simulink model "Variant1"  (R2021a)
settings: Solver=FixedStepAuto  StartTime=0.0  StopTime=STime  FixedStep=1e-3  RelTol=1e-3
undefined symbols (not defined in the file): C, J, Kp, Mc, Ra, Ta, Tp, Uc
settings Model: Creator=akangmufti  LastModifiedBy=akangmufti

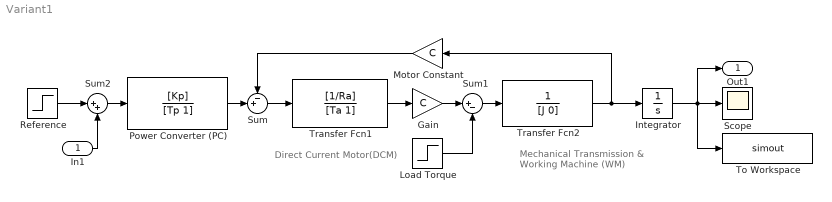
== system Variant1 ==
  note: Direct Current Motor(DCM)
  note: Mechanical Transmission &
      | Working Machine (WM)
  In1 : Inport
  Gain : Gain  Gain=C
  Integrator : Integrator  ContinuousStateAttributes='AngularPosition'
  Load Torque : Step  After=Mc  SampleTime=0
  Motor Constant : Gain  Gain=C
  Power Converter (PC) : TransferFcn  Numerator=[Kp]  Denominator=[Tp 1]
  Reference : Step  Time=1e-3  After=Uc  SampleTime=0
  Scope : Scope
  Sum : Sum  Inputs=-+|
  Sum1 : Sum  Inputs=|+-
  Sum2 : Sum  Inputs=|++
  To Workspace : ToWorkspace  VariableName=simout  SampleTime=1e-3
  Transfer Fcn1 : TransferFcn  Numerator=[1/Ra]  Denominator=[Ta 1]  ContinuousStateAttributes='Current'
  Transfer Fcn2 : TransferFcn  Denominator=[J 0]  ContinuousStateAttributes='Omega'
  Out1 : Outport
  wires:
  Motor Constant/1 -> Sum/1
  Power Converter (PC)/1 -> Sum/2
  Sum/1 -> Transfer Fcn1/1
  Transfer Fcn1/1 -> Gain/1
  Transfer Fcn2/1 -> Integrator/1, Motor Constant/1
  Integrator/1 -> Out1/1, To Workspace/1, Scope/1
  Sum1/1 -> Transfer Fcn2/1
  Gain/1 -> Sum1/1
  Load Torque/1 -> Sum1/2
  Reference/1 -> Sum2/1
  Sum2/1 -> Power Converter (PC)/1
  In1/1 -> Sum2/2
